simulink library "INT_CrC_DD"  (R2016b)
settings: Solver=VariableStepAuto  StartTime=0.0  StopTime=10.0  RelTol=1e-3
settings Model: Creator=xinchangran  LastModifiedBy=xinchangran

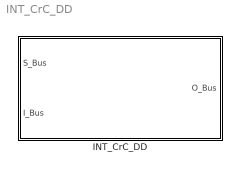
== system INT_CrC_DD ==
  INT_CrC_DD : Subsystem

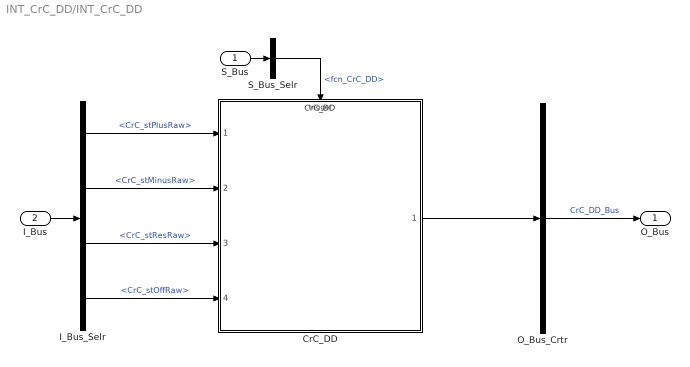
== system INT_CrC_DD/INT_CrC_DD ==
  S_Bus : Inport
  I_Bus : Inport  Port=2
  CrC_DD : ModelReference  ModelNameDialog=CrC_DD  SimulationMode=Normal  ModelReferenceVersion=1.39  TriggerPortName=function  TriggerPortTriggerType=function-call  TriggerPortStatesWhenEnabling=held
  I_Bus_Selr : BusSelector  OutputSignals=CrC_stPlusRaw,CrC_stMinusRaw,CrC_stResRaw,CrC_stOffRaw
  O_Bus_Crtr : BusCreator  Inputs=1
  S_Bus_Selr : BusSelector  OutputSignals=fcn_CrC_DD
  O_Bus : Outport
  wires:
  S_Bus_Selr/1 -> CrC_DD/Trigger  "<fcn_CrC_DD>"
  S_Bus/1 -> S_Bus_Selr/1
  I_Bus/1 -> I_Bus_Selr/1
  I_Bus_Selr/1 -> CrC_DD/1  "<CrC_stPlusRaw>"
  I_Bus_Selr/2 -> CrC_DD/2  "<CrC_stMinusRaw>"
  I_Bus_Selr/3 -> CrC_DD/3  "<CrC_stResRaw>"
  I_Bus_Selr/4 -> CrC_DD/4  "<CrC_stOffRaw>"
  O_Bus_Crtr/1 -> O_Bus/1  "CrC_DD_Bus"
  CrC_DD/1 -> O_Bus_Crtr/1
